simulink model "StateSpaceModel_withObserver_rev2"  (R2014b)
settings: Solver=ode45  StartTime=0.0  StopTime=10.0  RelTol=1e-3
values from neighbouring files (symbols this model uses):
  c1 = 0.01    [Variables_part2.m]
  c2 = 0.01    [Variables_part2.m]
  g = 9.81    [Variables_part2.m]
  J = M*L^2+m*l^2    (= 76.8)    [Variables_part2.m]
  k_bemf = 0.5    [Variables_part2.m]
  k_t = 0.75    [Variables_part2.m]
  L = 0.4    [Variables_part2.m]
  M = 55    [Variables_part2.m]
  m = 68    [Variables_part2.m]
  R = 0.5    [Variables_part2.m]
  r_a = 1.4    [Variables_part2.m]
settings Model: Creator=hchiang  LastModifiedBy=hchiang

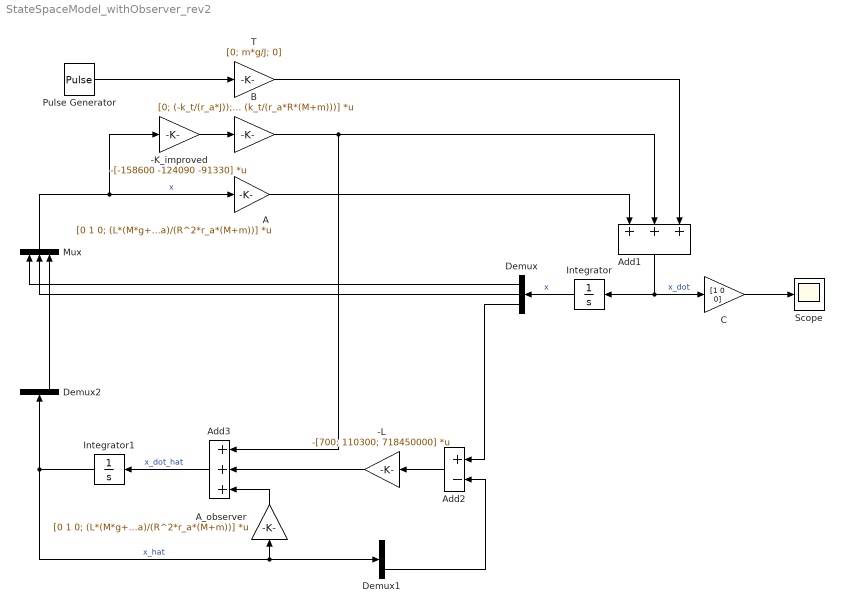
== system StateSpaceModel_withObserver_rev2 ==
  -K_improved : Gain  Gain=-[-158600 -124090 -91330]  Multiplication=Matrix(K*u)
  -L : Gain  Gain=-[700; 110300; 718450000]  Multiplication=Matrix(K*u)
  A : Gain  Gain=[0 1 0; (L*(M*g+m*g)/J) (-c1/J) (k_t*k_bemf/(R*r_a*J)); 0 0 -(k_t*k_bemf+c2*R^2*r_a)/(R^2*r_a*(M+m))]  Multiplication=Matrix(K*u)
  A_observer : Gain  Gain=[0 1 0; (L*(M*g+m*g)/J) (-c1/J) (k_t*k_bemf/(R*r_a*J)); 0 0 -(k_t*k_bemf+c2*R^2*r_a)/(R^2*r_a*(M+m))]  Multiplication=Matrix(K*u)
  Add1 : Sum  Inputs=+++
  Add2 : Sum  Inputs=+-
  Add3 : Sum  Inputs=+++
  B : Gain  Gain=[0; (-k_t/(r_a*J)); (k_t/(r_a*R*(M+m)))]  Multiplication=Matrix(K*u)
  C : Gain  Gain=[1 0 0]
  Demux : Demux  Outputs=3
  Demux1 : Demux  Outputs=3
  Demux2 : Demux  Outputs=3
  Integrator : Integrator
  Integrator1 : Integrator
  Mux : Mux  Inputs=3
  Pulse Generator : DiscretePulseGenerator  PulseType=Time based  Period=10  PulseWidth=5
  Scope : Scope
  T : Gain  Gain=[0; m*g/J; 0]
  wires:
  A/1 -> Add1/1
  Mux/1 -> -K_improved/1, A/1  "x"
  -K_improved/1 -> B/1
  B/1 -> Add1/2, Add3/1
  T/1 -> Add1/3
  Add1/1 -> C/1, Integrator/1  "x_dot"
  C/1 -> Scope/1
  Pulse Generator/1 -> T/1
  Integrator/1 -> Demux/1  "x"
  Demux/1 -> Mux/1
  Demux/2 -> Mux/2
  Add2/1 -> -L/1
  -L/1 -> Add3/2
  A_observer/1 -> Add3/3
  Add3/1 -> Integrator1/1  "x_dot_hat"
  Integrator1/1 -> Demux1/1, A_observer/1, Demux2/1  "x_hat"
  Demux1/3 -> Add2/2
  Demux/3 -> Add2/1
  Demux2/3 -> Mux/3
